simulink model "AION_signal_transfer"  (R2021a)
settings: configuration reference "AION_IDS_Speedgoat" (kept outside this file)
libraries: simulink x1
settings Model: DataDictionary=AION_IDS.sldd  Creator=xinrui  LastModifiedBy=Administrator
settings ConfigSetRef: SourceName=AION_IDS_Speedgoat

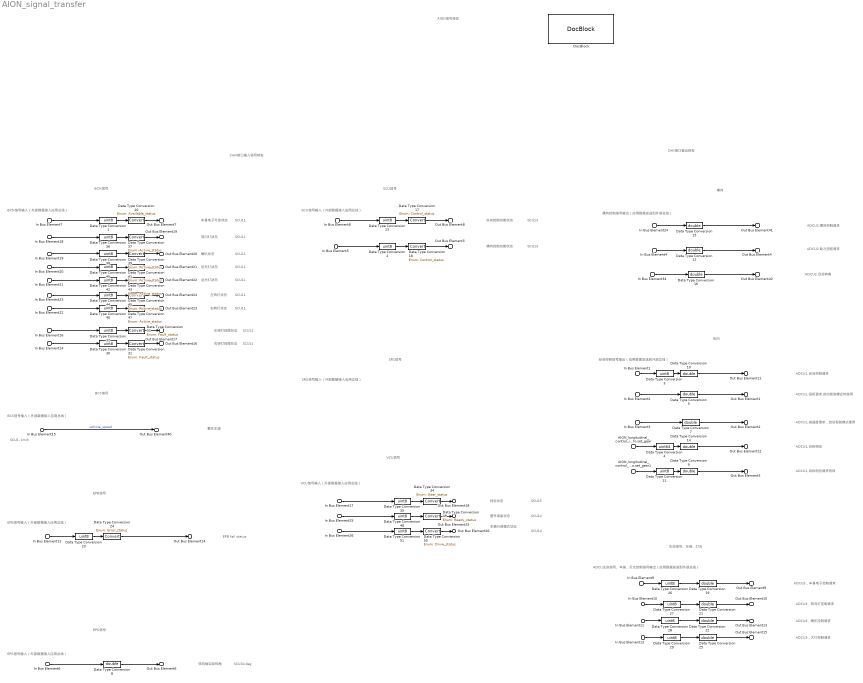
== system AION_signal_transfer ==
  note: AION信号转发
  note: 纵向控制信号输出（应用数据发送到外部总线）
  note: ADCU2,目标转角
  note: 整车车速
  note: ADCU1,目标档位
  note: SCU信号输入（外部数据接入应用总线）
  note: 横向控制信号输出（应用数据发送到外部总线）
  note: ADCU2,横向控制请求
  note: ADCU1,纵向控制请求
  note: CAN接口输入信号转发
  note: SCU13
  note: SCU1, km/h
  note: ADCU1,扭矩请求,自动驾驶模式时使用
  note: ADCU1,减速度请求，自动驾驶模式使用
  note: ADCU1,目标档位请求有效
  note: SCU13
  note: SCU10,deg
  note: 横向控制功能状态
  note: SRS信号输入（外部数据接入应用总线）
  note: 转向轴实际转角
  note: BCM信号输入（外部数据接入应用总线）
  note: 纵向控制功能状态
  note: ADCU生命信号、车身、灯光控制信号输出（应用数据发送到外部总线）
  note: ADCU2,助力扭矩请求
  note: BCS信号输入（外部数据接入应用总线）
  note: EPB信号输入（外部数据接入应用总线）
  note: EPS信号输入（外部数据接入应用总线）
  note: VCU信号输入（外部数据接入应用总线）
  note: EPB fail status
  note: ADCU3，车身电子控制请求
  note: ADCU3，转向灯控制请求
  note: ADCU3，喇叭控制请求
  note: ADCU3，大灯控制请求
  note: CAN接口输出转发
  note: BCS信号
  note: BCM信号
  note: EPB信号
  note: EPS信号
  note: SCU信号
  note: SRS信号
  note: VCU信号
  note: 纵向
  note: 横向
  note: 生命信号、车身、灯光
  note: SCU15
  note: 挡位状态
  note: 车身电子可控状态
  note: SCU11
  note: 双闪灯状态
  note: SCU11
  note: SCU11
  note: SCU11
  note: SCU11
  note: SCU11
  note: 喇叭状态
  note: 近光灯状态
  note: 远光灯状态
  note: SCU11
  note: 左转灯故障状态
  note: 右转灯故障状态
  note: SCU11
  note: 左转灯状态
  note: 右转灯状态
  note: SCU11
  note: 整车准备状态
  note: 车辆行驶模式状态
  note: SCU14
  note: SCU14
  In Bus Element15 : Inport  PortName=ADCU_InputPort  Element=InputCAN_bus.SCU2ADCU_bus.SCU_1.BCS_VehSpd
  In Bus Element6 : Inport  PortName=ADCU_InputPort  Element=InputCAN_bus.SCU2ADCU_bus.SCU_10.EPS_SteeringAngle
  In Bus Element7 : Inport  PortName=ADCU_InputPort  Element=InputCAN_bus.SCU2ADCU_bus.SCU_11.BCM_CtrlAvailable
  In Bus Element18 : Inport  PortName=ADCU_InputPort  Element=InputCAN_bus.SCU2ADCU_bus.SCU_11.BCM_HazardLampSt
  In Bus Element21 : Inport  PortName=ADCU_InputPort  Element=InputCAN_bus.SCU2ADCU_bus.SCU_11.BCM_HighBeamSt
  In Bus Element19 : Inport  PortName=ADCU_InputPort  Element=InputCAN_bus.SCU2ADCU_bus.SCU_11.BCM_HornSt
  In Bus Element16 : Inport  PortName=ADCU_InputPort  Element=InputCAN_bus.SCU2ADCU_bus.SCU_11.BCM_LeftTurnLampFaultSt
  In Bus Element23 : Inport  PortName=ADCU_InputPort  Element=InputCAN_bus.SCU2ADCU_bus.SCU_11.BCM_LeftTurnLampSt
  In Bus Element20 : Inport  PortName=ADCU_InputPort  Element=InputCAN_bus.SCU2ADCU_bus.SCU_11.BCM_LowBeamSt
  In Bus Element14 : Inport  PortName=ADCU_InputPort  Element=InputCAN_bus.SCU2ADCU_bus.SCU_11.BCM_RightTurnLampFaultSt
  In Bus Element22 : Inport  PortName=ADCU_InputPort  Element=InputCAN_bus.SCU2ADCU_bus.SCU_11.BCM_RightTurnLampSt
  In Bus Element5 : Inport  PortName=ADCU_InputPort  Element=InputCAN_bus.SCU2ADCU_bus.SCU_13.SCU_LatCtrlMode
  In Bus Element8 : Inport  PortName=ADCU_InputPort  Element=InputCAN_bus.SCU2ADCU_bus.SCU_13.SCU_LngCtrlMode
  In Bus Element26 : Inport  PortName=ADCU_InputPort  Element=InputCAN_bus.SCU2ADCU_bus.SCU_14.VCU_VehDrvMod
  In Bus Element25 : Inport  PortName=ADCU_InputPort  Element=InputCAN_bus.SCU2ADCU_bus.SCU_14.VCU_VehRdySt
  In Bus Element17 : Inport  PortName=ADCU_InputPort  Element=InputCAN_bus.SCU2ADCU_bus.SCU_15.VCU_CrntGearLvl
  In Bus Element12 : Inport  PortName=ADCU_InputPort  Element=InputCAN_bus.SCU2ADCU_bus.SCU_9.EPB_FailSt
  In Bus Element24 : Inport  Port=2  PortName=ADCU_InternalOutputPort  Element=set_lateral_control_info.set_LatCtrlReq
  In Bus Element4 : Inport  Port=2  PortName=ADCU_InternalOutputPort  Element=set_lateral_control_info.set_SteerWhlTorqReq
  In Bus Element34 : Inport  Port=2  PortName=ADCU_InternalOutputPort  Element=set_lateral_control_info.set_SteerAngReq
  In Bus Element1 : Inport  Port=2  PortName=ADCU_InternalOutputPort  Element=set_longitudinal_control_info.set_LngCtrlReq
  In Bus Element2 : Inport  Port=2  PortName=ADCU_InternalOutputPort  Element=set_longitudinal_control_info.set_AutoTrqWhlReq
  In Bus Element3 : Inport  Port=2  PortName=ADCU_InternalOutputPort  Element=set_longitudinal_control_info.set_BrakeReq
  AION_longitudinal_control_info.set_gear : Inport  Port=2  PortName=ADCU_InternalOutputPort  Element=set_longitudinal_control_info.set_GearLvlReq
  AION_longitudinal_control_info.set_gear1 : Inport  Port=2  PortName=ADCU_InternalOutputPort  Element=set_longitudinal_control_info.set_GearLvlReqVD
  In Bus Element13 : Inport  Port=2  PortName=ADCU_InternalOutputPort  Element=set_ADCU_info.set_BeamReq
  In Bus Element9 : Inport  Port=2  PortName=ADCU_InternalOutputPort  Element=set_ADCU_info.set_BodyCtrlReq
  In Bus Element11 : Inport  Port=2  PortName=ADCU_InternalOutputPort  Element=set_ADCU_info.set_HornRingReq
  In Bus Element10 : Inport  Port=2  PortName=ADCU_InternalOutputPort  Element=set_ADCU_info.set_TurnLightReq
  Data Type Conversion{1..3,11,13,23,26..30,32,35..36,38,40,42,44,46,48,51} (21 alike) : DataTypeConversion  OutDataTypeStr=uint8
  Data Type Conversion{5,7..10,12,14..16,19,21..22,25} (13 alike) : DataTypeConversion  OutDataTypeStr=double
  Data Type Conversion17 : DataTypeConversion  OutDataTypeStr=Enum: Control_status
  Data Type Conversion18 : DataTypeConversion  OutDataTypeStr=Enum: Control_status
  Data Type Conversion20 : DataTypeConversion  OutDataTypeStr=Enum: Available_status
  Data Type Conversion24 : DataTypeConversion  OutDataTypeStr=Enum: Error_status
  Data Type Conversion31 : DataTypeConversion  OutDataTypeStr=Enum: Fault_status
  Data Type Conversion33 : DataTypeConversion  OutDataTypeStr=Enum: Fault_status
  Data Type Conversion34 : DataTypeConversion  OutDataTypeStr=Enum: Gear_status
  Data Type Conversion{37,39,41,43,45,47} (6 alike) : DataTypeConversion  OutDataTypeStr=Enum: Active_status
  Data Type Conversion4 : DataTypeConversion  OutDataTypeStr=uint64
  Data Type Conversion49 : DataTypeConversion  OutDataTypeStr=Enum: Ready_status
  Data Type Conversion50 : DataTypeConversion  OutDataTypeStr=Enum: Drive_status
  DocBlock : simulink/Model-Wide Utilities/DocBlock  DocumentType=HTML  mask(DocBlock){}
      mask Display:
      | plot([.8 0 0 1 1 .8 .8 1],[1 1 0 0 .8 1 .8 .8]);
      | text(.5,.6,'CHANGELOG','horizontalalignment','center');
      | text(.95,.05,get_param(gcb,'DocumentType'),'verticalalignment','bottom','horizontalalignment','right');
  Out Bus Element40 : Outport  PortName=ADCU_InternalInputPort  Element=get_BCS_info.get_VehSpd
  Out Bus Element26 : Outport  PortName=ADCU_InternalInputPort  Element=get_VCU_info.get_VehDrvMod
  Out Bus Element25 : Outport  PortName=ADCU_InternalInputPort  Element=get_VCU_info.get_VehRdySt
  Out Bus Element18 : Outport  PortName=ADCU_InternalInputPort  Element=get_VCU_info.get_CrntGearLvl
  Out Bus Element5 : Outport  PortName=ADCU_InternalInputPort  Element=get_SCU_info.get_LatCtrlMode
  Out Bus Element8 : Outport  PortName=ADCU_InternalInputPort  Element=get_SCU_info.get_LngCtrlMode
  Out Bus Element14 : Outport  PortName=ADCU_InternalInputPort  Element=get_EPB_info.get_FailSt
  Out Bus Element6 : Outport  PortName=ADCU_InternalInputPort  Element=get_EPS_info.get_SteeringAngle
  Out Bus Element7 : Outport  PortName=ADCU_InternalInputPort  Element=get_BCM_info.get_CtrlAvailable
  Out Bus Element19 : Outport  PortName=ADCU_InternalInputPort  Element=get_BCM_info.get_HazardLampSt
  Out Bus Element22 : Outport  PortName=ADCU_InternalInputPort  Element=get_BCM_info.get_HighBeamSt
  Out Bus Element20 : Outport  PortName=ADCU_InternalInputPort  Element=get_BCM_info.get_HornSt
  Out Bus Element17 : Outport  PortName=ADCU_InternalInputPort  Element=get_BCM_info.get_LeftTurnLampFaultSt
  Out Bus Element24 : Outport  PortName=ADCU_InternalInputPort  Element=get_BCM_info.get_LeftTurnLampSt
  Out Bus Element21 : Outport  PortName=ADCU_InternalInputPort  Element=get_BCM_info.get_LowBeamSt
  Out Bus Element16 : Outport  PortName=ADCU_InternalInputPort  Element=get_BCM_info.get_RightTurnLampFaultSt
  Out Bus Element23 : Outport  PortName=ADCU_InternalInputPort  Element=get_BCM_info.get_RightTurnLampSt
  Out Bus Element1 : Outport  Port=2  PortName=ADCU_OuputPort  Element=OutputCAN_bus.ADCU2SCU_bus.ADCU_1.ADCU_AutoTrqWhlReq
  Out Bus Element2 : Outport  Port=2  PortName=ADCU_OuputPort  Element=OutputCAN_bus.ADCU2SCU_bus.ADCU_1.ADCU_BrakeReq
  Out Bus Element12 : Outport  Port=2  PortName=ADCU_OuputPort  Element=OutputCAN_bus.ADCU2SCU_bus.ADCU_1.ADCU_GearLvlReq
  Out Bus Element3 : Outport  Port=2  PortName=ADCU_OuputPort  Element=OutputCAN_bus.ADCU2SCU_bus.ADCU_1.ADCU_GearLvlReqVD
  Out Bus Element11 : Outport  Port=2  PortName=ADCU_OuputPort  Element=OutputCAN_bus.ADCU2SCU_bus.ADCU_1.ADCU_LngCtrlReq
  Out Bus Element41 : Outport  Port=2  PortName=ADCU_OuputPort  Element=OutputCAN_bus.ADCU2SCU_bus.ADCU_2.ADCU_LatCtrlReq
  Out Bus Element42 : Outport  Port=2  PortName=ADCU_OuputPort  Element=OutputCAN_bus.ADCU2SCU_bus.ADCU_2.ADCU_SteerAngReq
  Out Bus Element4 : Outport  Port=2  PortName=ADCU_OuputPort  Element=OutputCAN_bus.ADCU2SCU_bus.ADCU_2.ADCU_SteerWhlTorqReq
  Out Bus Element15 : Outport  Port=2  PortName=ADCU_OuputPort  Element=OutputCAN_bus.ADCU2SCU_bus.ADCU_3.ADCU_BeamReq
  Out Bus Element9 : Outport  Port=2  PortName=ADCU_OuputPort  Element=OutputCAN_bus.ADCU2SCU_bus.ADCU_3.ADCU_BodyCtrlReq
  Out Bus Element13 : Outport  Port=2  PortName=ADCU_OuputPort  Element=OutputCAN_bus.ADCU2SCU_bus.ADCU_3.ADCU_HornRingReq
  Out Bus Element10 : Outport  Port=2  PortName=ADCU_OuputPort  Element=OutputCAN_bus.ADCU2SCU_bus.ADCU_3.ADCU_TurnLightReq
  wires:
  In Bus Element15/1 -> Out Bus Element40/1  "vehicle_speed"
  In Bus Element1/1 -> Data Type Conversion3/1
  Data Type Conversion10/1 -> Out Bus Element11/1
  Data Type Conversion14/1 -> Out Bus Element12/1
  In Bus Element24/1 -> Data Type Conversion15/1
  Data Type Conversion15/1 -> Out Bus Element41/1
  Data Type Conversion16/1 -> Out Bus Element42/1
  In Bus Element34/1 -> Data Type Conversion16/1
  Data Type Conversion3/1 -> Data Type Conversion10/1
  AION_longitudinal_control_info.set_gear/1 -> Data Type Conversion4/1
  Data Type Conversion5/1 -> Out Bus Element1/1
  In Bus Element3/1 -> Data Type Conversion7/1
  Data Type Conversion9/1 -> Out Bus Element3/1
  AION_longitudinal_control_info.set_gear1/1 -> Data Type Conversion11/1
  Data Type Conversion11/1 -> Data Type Conversion9/1
  In Bus Element4/1 -> Data Type Conversion12/1
  Data Type Conversion12/1 -> Out Bus Element4/1
  Data Type Conversion2/1 -> Data Type Conversion18/1
  In Bus Element6/1 -> Data Type Conversion8/1
  In Bus Element5/1 -> Data Type Conversion2/1
  Data Type Conversion18/1 -> Out Bus Element5/1
  Data Type Conversion17/1 -> Out Bus Element8/1
  Data Type Conversion13/1 -> Data Type Conversion17/1
  In Bus Element8/1 -> Data Type Conversion13/1
  Data Type Conversion1/1 -> Data Type Conversion20/1
  In Bus Element7/1 -> Data Type Conversion1/1
  Data Type Conversion20/1 -> Out Bus Element7/1
  In Bus Element12/1 -> Data Type Conversion23/1
  Data Type Conversion23/1 -> Data Type Conversion24/1
  Data Type Conversion24/1 -> Out Bus Element14/1
  Data Type Conversion4/1 -> Data Type Conversion14/1
  Data Type Conversion19/1 -> Out Bus Element9/1
  In Bus Element9/1 -> Data Type Conversion26/1
  In Bus Element10/1 -> Data Type Conversion27/1
  Data Type Conversion21/1 -> Out Bus Element10/1
  In Bus Element11/1 -> Data Type Conversion28/1
  Data Type Conversion22/1 -> Out Bus Element13/1
  In Bus Element13/1 -> Data Type Conversion29/1
  Data Type Conversion25/1 -> Out Bus Element15/1
  Data Type Conversion26/1 -> Data Type Conversion19/1
  Data Type Conversion27/1 -> Data Type Conversion21/1
  Data Type Conversion28/1 -> Data Type Conversion22/1
  Data Type Conversion29/1 -> Data Type Conversion25/1
  Data Type Conversion31/1 -> Out Bus Element16/1
  In Bus Element14/1 -> Data Type Conversion30/1
  Data Type Conversion30/1 -> Data Type Conversion31/1
  Data Type Conversion33/1 -> Out Bus Element17/1
  Data Type Conversion32/1 -> Data Type Conversion33/1
  In Bus Element16/1 -> Data Type Conversion32/1
  In Bus Element2/1 -> Data Type Conversion5/1
  In Bus Element17/1 -> Data Type Conversion35/1
  Data Type Conversion35/1 -> Data Type Conversion34/1
  Data Type Conversion34/1 -> Out Bus Element18/1
  Data Type Conversion37/1 -> Out Bus Element19/1
  In Bus Element18/1 -> Data Type Conversion36/1
  Data Type Conversion36/1 -> Data Type Conversion37/1
  Data Type Conversion38/1 -> Data Type Conversion39/1
  In Bus Element19/1 -> Data Type Conversion38/1
  Data Type Conversion39/1 -> Out Bus Element20/1
  Data Type Conversion41/1 -> Out Bus Element21/1
  In Bus Element20/1 -> Data Type Conversion40/1
  Data Type Conversion40/1 -> Data Type Conversion41/1
  Data Type Conversion42/1 -> Data Type Conversion43/1
  In Bus Element21/1 -> Data Type Conversion42/1
  Data Type Conversion43/1 -> Out Bus Element22/1
  Data Type Conversion47/1 -> Out Bus Element23/1
  In Bus Element22/1 -> Data Type Conversion46/1
  Data Type Conversion46/1 -> Data Type Conversion47/1
  Data Type Conversion44/1 -> Data Type Conversion45/1
  In Bus Element23/1 -> Data Type Conversion44/1
  Data Type Conversion45/1 -> Out Bus Element24/1
  In Bus Element25/1 -> Data Type Conversion48/1
  Data Type Conversion48/1 -> Data Type Conversion49/1
  In Bus Element26/1 -> Data Type Conversion51/1
  Data Type Conversion51/1 -> Data Type Conversion50/1
  Data Type Conversion50/1 -> Out Bus Element26/1
  Data Type Conversion49/1 -> Out Bus Element25/1
  Data Type Conversion7/1 -> Out Bus Element2/1
  Data Type Conversion8/1 -> Out Bus Element6/1
